simulink model "Motor1Response"  (R2017a)
settings: Solver=VariableStepAuto  StartTime=0.0  StopTime=1  RelTol=1e-3
undefined symbols (not defined in the file or in its folder): Elec1d, Elec1n, Mech1d, Mech1n, SpdCon1, TCon1
libraries: simulink x1
settings Model: Creator=Matthew  LastModifiedBy=Matthew

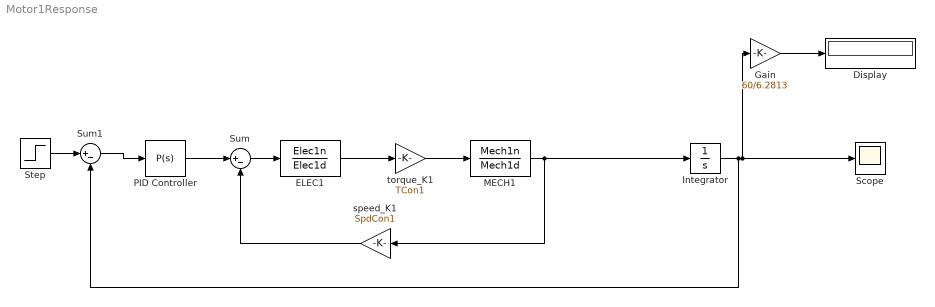
== system Motor1Response ==
  Display : Display
  "ELEC1 " : TransferFcn  Numerator=Elec1n  Denominator=Elec1d
  Gain : Gain  Gain=60/6.2813
  Integrator : Integrator
  "MECH1 " : TransferFcn  Numerator=Mech1n  Denominator=Mech1d
  PID Controller : simulink/Continuous/PID Controller  Controller=P  TimeDomain=Continuous-time  SampleTime=-1  IntegratorMethod=Forward Euler  FilterMethod=Forward Euler  Form=Parallel  UseFilter=on  ControllerParametersSource=internal  P=1  I=1  D=1  N=100  InitialConditionSource=internal  InitialConditionForIntegrator=0  InitialConditionForFilter=0  ExternalReset=none  LimitOutput=off  UpperSaturationLimit=inf  LowerSaturationLimit=-inf  LinearizeAsGain=on  AntiWindupMode=none  Kb=1  TrackingMode=off  Kt=1  PParamMin=[]  PParamMax=[]  IParamMin=[]  IParamMax=[]  DParamMin=[]  DParamMax=[]  NParamMin=[]  NParamMax=[]  KbParamMin=[]  KbParamMax=[]  KtParamMin=[]  KtParamMax=[]  POutMin=[]  POutMax=[]  IOutMin=[]  IOutMax=[]  DOutMin=[]  DOutMax=[]  NOutMin=[]  NOutMax=[]  KbOutMin=[]  KbOutMax=[]  KtOutMin=[]  KtOutMax=[]  IntegratorOutMin=[]  IntegratorOutMax=[]  FilterOutMin=[]  FilterOutMax=[]  SumOutMin=[]  SumOutMax=[]  SumI1OutMin=[]  SumI1OutMax=[]  SumI2OutMin=[]  SumI2OutMax=[]  SumI3OutMin=[]  SumI3OutMax=[]  SumDOutMin=[]  SumDOutMax=[]  SaturationOutMin=[]  SaturationOutMax=[]  IntegratorContinuousStateAttributes=''  IntegratorStateMustResolveToSignalObject=off  IntegratorRTWStateStorageClass=Auto  FilterContinuousStateAttributes=''  FilterStateMustResolveToSignalObject=off  FilterRTWStateStorageClass=Auto  DifferentiatorICPrevScaledInput=0  DifferentiatorOutMin=[]  DifferentiatorOutMax=[]  InitialConditionSetting=State (most efficient)
  Scope : Scope
  Step : Step  Time=0  SampleTime=0
  Sum : Sum  Inputs=|+-
  Sum1 : Sum  Inputs=|+-
  speed_K1 : Gain  Gain=SpdCon1
  "torque_K1 " : Gain  Gain=TCon1
  wires:
  speed_K1/1 -> Sum/2
  "torque_K1 "/1 -> "MECH1 "/1
  Sum/1 -> "ELEC1 "/1
  "ELEC1 "/1 -> "torque_K1 "/1
  "MECH1 "/1 -> Integrator/1, speed_K1/1
  Gain/1 -> Display/1
  PID Controller/1 -> Sum/1
  Integrator/1 -> Sum1/2, Gain/1, Scope/1
  Step/1 -> Sum1/1
  Sum1/1 -> PID Controller/1
